simulink model "quadrotor_system_observer"  (R2022a)
settings: Solver=VariableStepAuto  StartTime=0.0  StopTime=70  RelTol=1e-3
values from neighbouring files (symbols this model uses):
  A1 = [-skew(Oc) ,eye(3),-skew(Vc),zeros(3),zeros(3,4) ... (first row only)    [controllerLinearizedSystemScript.m]
  B1 = [[0;0;0],zeros(3) ... (first row only)    [controllerLinearizedSystemScript.m]
  C1 = [eye(3), zeros(3), zeros(3), zeros(3), zeros(3,4) ... (first row only)    [controllerLinearizedSystemScript.m]
  K1 = lqr(A1,B1,Q1,R1,0)    [controllerLinearizedSystemScript.m]
undefined symbols (not defined in the file or in its folder): L
libraries: robotcorelib x1, uavutilslib x1
settings Model: PacingRate=4  Creator=Lenovo  LastModifiedBy=FLKU

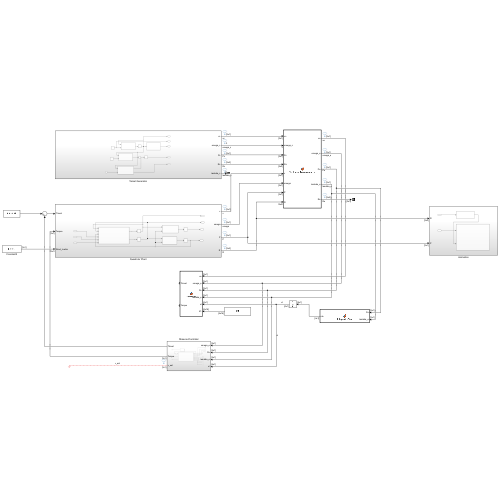
[thumbnail: Simulink's stored preview of the top-level diagram]
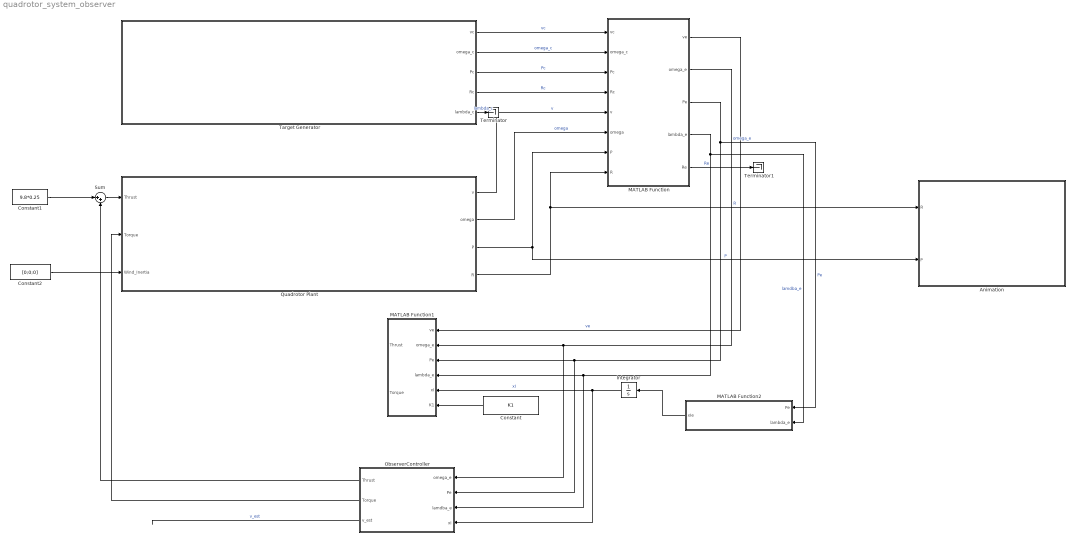
== system quadrotor_system_observer ==
  Animation : Subsystem
  Constant : Constant  Value=K1
  Constant1 : Constant  Value=9.8*0.25
  Constant2 : Constant  Value=[0;0;0]  VectorParams1D=off  SampleTime=-1
  Integrator : Integrator
  MATLAB Function : MATLAB Function  TreatAsAtomicUnit=on
  MATLAB Function1 : MATLAB Function  TreatAsAtomicUnit=on
  MATLAB Function2 : MATLAB Function  TreatAsAtomicUnit=on
  ObserverController : Subsystem
  Quadrotor Plant : Subsystem
  Sum : Sum  Inputs=|++
  Target Generator : Subsystem
  Terminator : Terminator
  Terminator1 : Terminator
  wires:
  Target Generator/1(vc) -> MATLAB Function/1(vc)  "vc"
  Target Generator/2(omega_c) -> MATLAB Function/2(omega_c)  "omega_c"
  Target Generator/3(Pc) -> MATLAB Function/3(Pc)  "Pc"
  Target Generator/4(Rc) -> MATLAB Function/4(Rc)  "Rc"
  Quadrotor Plant/4(R) -> MATLAB Function/8(R), Animation/1(R)  "R"
  Quadrotor Plant/3(P) -> Animation/2(P), MATLAB Function/7(P)  "P"
  Quadrotor Plant/2(omega) -> MATLAB Function/6(omega)  "omega"
  Quadrotor Plant/1(v) -> MATLAB Function/5(v)  "v"
  MATLAB Function/4(lambda_e) -> ObserverController/3(lamdba_e), MATLAB Function1/4(lambda_e), MATLAB Function2/2(lambda_e)  "lamdba_e"
  MATLAB Function/3(Pe) -> MATLAB Function1/3(Pe), ObserverController/2(Pe), MATLAB Function2/1(Pe)  "Pe"
  MATLAB Function/2(omega_e) -> MATLAB Function1/2(omega_e), ObserverController/1(omega_e)  "omega_e"
  MATLAB Function/1(ve) -> MATLAB Function1/1(ve)  "ve"
  Target Generator/5(lambda_c) -> Terminator/1  "lambda_c"
  Constant/1 -> MATLAB Function1/6(K1)
  Sum/1 -> Quadrotor Plant/1(Thrust)
  Constant1/1 -> Sum/1
  Constant2/1 -> Quadrotor Plant/3(Wind_Inertia)
  MATLAB Function2/1(xIe) -> Integrator/1
  Integrator/1 -> ObserverController/4(xI), MATLAB Function1/5(xI)  "xI"
  MATLAB Function/5(Re) -> Terminator1/1  "Re"
  ObserverController/3(v_est) -> ?  "v_est"
  ObserverController/1(Thrust) -> Sum/2
  ObserverController/2(Torque) -> Quadrotor Plant/2(Torque)

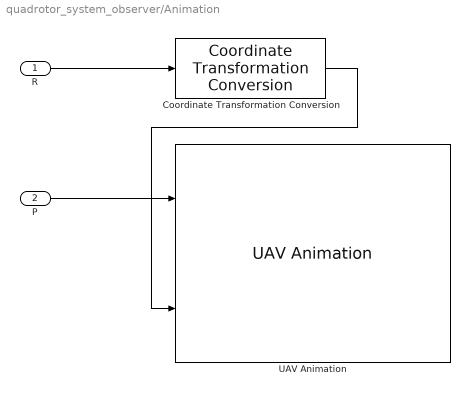
== system quadrotor_system_observer/Animation ==
  R : Inport
  P : Inport  Port=2
  Coordinate Transformation Conversion : robotcorelib/Coordinate Transformation Conversion  InputRepresentation=Rotation Matrix  InputEulerSequence=ZYX  ShowTrVecInputPort=on  OutputRepresentation=Quaternion  OutputEulerSequence=ZYX  ShowTrVecOutputPort=on  SimulateUsing=Interpreted execution
      settings: SourceProductBaseCode=RO,NV,RR,UV
  UAV Animation : uavutilslib/UAV Animation  UAVType=Multirotor  UAVSize=1  InertialZDirection=Down  SampleTime=-1
      settings: SourceProductBaseCode=UV
  wires:
  Coordinate Transformation Conversion/1 -> UAV Animation/2
  P/1 -> UAV Animation/1
  R/1 -> Coordinate Transformation Conversion/1

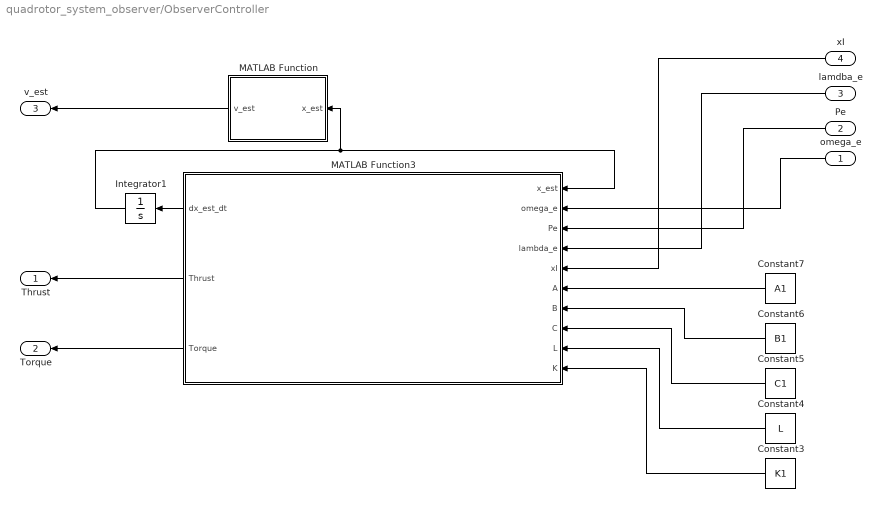
== system quadrotor_system_observer/ObserverController ==
  omega_e : Inport
  Pe : Inport  Port=2
  lamdba_e : Inport  Port=3
  xI : Inport  Port=4
  Constant3 : Constant  Value=K1
  Constant4 : Constant  Value=L
  Constant5 : Constant  Value=C1
  Constant6 : Constant  Value=B1
  Constant7 : Constant  Value=A1
  Integrator1 : Integrator  InitialCondition=zeros(16,1)
  MATLAB Function : MATLAB Function  TreatAsAtomicUnit=on
  MATLAB Function3 : MATLAB Function  TreatAsAtomicUnit=on
  Thrust : Outport
  Torque : Outport  Port=2
  v_est : Outport  Port=3
  wires:
  Constant7/1 -> MATLAB Function3/6(A)
  MATLAB Function3/3(Torque) -> Torque/1
  Constant4/1 -> MATLAB Function3/9(L)
  Integrator1/1 -> MATLAB Function/1(x_est), MATLAB Function3/1(x_est)
  Constant6/1 -> MATLAB Function3/7(B)
  Constant3/1 -> MATLAB Function3/10(K)
  MATLAB Function3/1(dx_est_dt) -> Integrator1/1
  Constant5/1 -> MATLAB Function3/8(C)
  MATLAB Function3/2(Thrust) -> Thrust/1
  xI/1 -> MATLAB Function3/5(xI)
  omega_e/1 -> MATLAB Function3/2(omega_e)
  Pe/1 -> MATLAB Function3/3(Pe)
  lamdba_e/1 -> MATLAB Function3/4(lambda_e)
  MATLAB Function/1(v_est) -> v_est/1

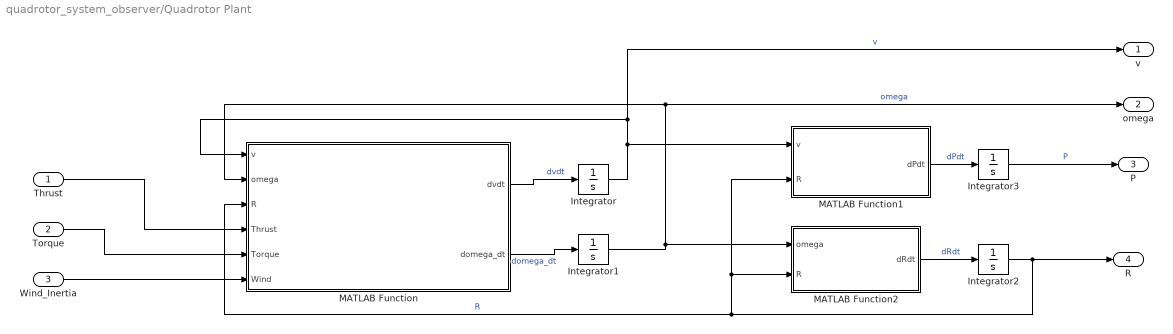
== system quadrotor_system_observer/Quadrotor Plant ==
  Thrust : Inport
  Torque : Inport  Port=2
  Wind_Inertia : Inport  Port=3
  Integrator : Integrator  InitialCondition=[0;0;0]
  Integrator1 : Integrator  InitialCondition=[0;0;0]
  Integrator2 : Integrator  InitialCondition=eye(3)
  Integrator3 : Integrator  InitialCondition=[0;0;0]
  MATLAB Function : MATLAB Function  TreatAsAtomicUnit=on
  MATLAB Function1 : MATLAB Function  TreatAsAtomicUnit=on
  MATLAB Function2 : MATLAB Function  TreatAsAtomicUnit=on
  v : Outport
  omega : Outport  Port=2
  P : Outport  Port=3
  R : Outport  Port=4
  wires:
  Integrator2/1 -> R/1, MATLAB Function/3(R), MATLAB Function2/2(R), MATLAB Function1/2(R)  "R"
  MATLAB Function/1(dvdt) -> Integrator/1  "dvdt"
  Integrator1/1 -> MATLAB Function2/1(omega), MATLAB Function/2(omega), omega/1  "omega"
  MATLAB Function/2(domega_dt) -> Integrator1/1  "domega_dt"
  Thrust/1 -> MATLAB Function/4(Thrust)
  MATLAB Function1/1(dPdt) -> Integrator3/1  "dPdt"
  Integrator3/1 -> P/1  "P"
  MATLAB Function2/1(dRdt) -> Integrator2/1  "dRdt"
  Integrator/1 -> v/1, MATLAB Function/1(v), MATLAB Function1/1(v)  "v"
  Torque/1 -> MATLAB Function/5(Torque)
  Wind_Inertia/1 -> MATLAB Function/6(Wind)

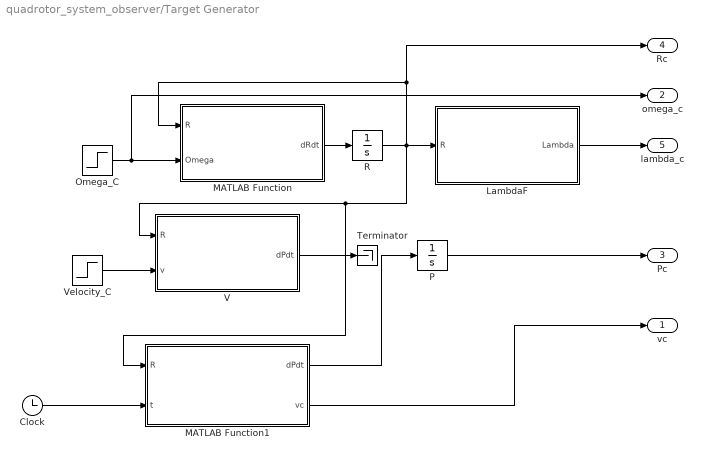
== system quadrotor_system_observer/Target Generator ==
  Clock : Clock
  LambdaF : MATLAB Function  TreatAsAtomicUnit=on
  MATLAB Function : MATLAB Function  TreatAsAtomicUnit=on
  MATLAB Function1 : MATLAB Function  TreatAsAtomicUnit=on
  Omega_C : Step  Time=0  Before=[0;0;0]  After=[0;0;0]  SampleTime=0
  P : Integrator  InitialCondition=[0;0;0]
  R : Integrator  InitialCondition=eye(3)
  Terminator : Terminator
  V : MATLAB Function  TreatAsAtomicUnit=on
  Velocity_C : Step  Time=0  Before=[0;0;0]  After=[2;0;0]  SampleTime=0
  vc : Outport
  omega_c : Outport  Port=2
  Pc : Outport  Port=3
  Rc : Outport  Port=4
  lambda_c : Outport  Port=5
  wires:
  LambdaF/1(Lambda) -> lambda_c/1
  P/1 -> Pc/1
  MATLAB Function/1(dRdt) -> R/1
  R/1 -> MATLAB Function/1(R), Rc/1, MATLAB Function1/1(R), V/1(R), LambdaF/1(R)
  Velocity_C/1 -> V/2(v)
  Omega_C/1 -> omega_c/1, MATLAB Function/2(Omega)
  Clock/1 -> MATLAB Function1/2(t)
  MATLAB Function1/1(dPdt) -> P/1
  MATLAB Function1/2(vc) -> vc/1
  V/1(dPdt) -> Terminator/1

== matlab function quadrotor_system_observer/MATLAB Function2 ==
  data: Pe input; xIe output; lambda_e input
function xIe = IntegrationVar(Pe,lambda_e)

xIe = [Pe;lambda_e(3)];

== matlab function quadrotor_system_observer/ObserverController/MATLAB Function3 ==
  data: x_est input; omega_e input; dx_est_dt output; Pe input; lambda_e input; xI input; A input; B input; C input; L input; K input; Thrust output; Torque output
function [dx_est_dt,Thrust,Torque]   = observer_controller(x_est,omega_e,Pe,lambda_e,xI,A,B,C,L,K)
%% controller
u = -K*x_est;
Thrust=u(1);
Torque=u(2:4);
%% observer
y=[Pe;lambda_e;omega_e;xI];
dx_est_dt = (A-L*C)*x_est+L*y+B*u;
end

== matlab function quadrotor_system_observer/Target Generator/MATLAB Function1 ==
  data: R input; t input; dPdt output; vc output
function [dPdt,vc] = GenRecTrajVc(R,t)
v = 0.5;
vc = [0;0;0];
if t>5
    vc = [v;0;0];
end
if t>15
    vc = [0;0;0];
end
if t>20
    vc = [0;v;0];
end
if t>30
    vc = [0;0;0];
end
if t>35
    vc = [-v;0;0];
end
if t>45
    vc = [0;0;0];
end
if t>50
    vc = [0;-v;0];
end
dPdt = R*vc;
end

== matlab function quadrotor_system_observer/ObserverController/MATLAB Function ==
  data: x_est input; v_est output
function v_est = chooseVEstima(x_est)

v_est = x_est(4:6);

== matlab function quadrotor_system_observer/Quadrotor Plant/MATLAB Function1 ==
  data: v input; dPdt output; R input
function dPdt = TranslationalKinematics(v,R)
dPdt = R*v;

== matlab function quadrotor_system_observer/Quadrotor Plant/MATLAB Function ==
  data: v input; omega input; R input; Thrust input; dvdt output; Torque input; domega_dt output; Wind input
function [dvdt, domega_dt] = Dynamics(v,omega,R,Thrust, Torque, Wind)
g = 9.807;
m = 0.24;
f_B = [0;0;-Thrust] + transpose(R) * [0;0;m*g] + transpose(R) * Wind;
I_B = diag([1e-4,1e-4,1e-3]);

dvdt = -skew(omega) * v + 1/m * f_B;
domega_dt = -(I_B^-1) * skew(omega) * I_B * omega + (I_B^-1) * Torque;
end

== matlab function quadrotor_system_observer/Quadrotor Plant/MATLAB Function2 ==
  data: omega input; dRdt output; R input
function dRdt = RotationalKinematics(omega,R)
dRdt = R*skew(omega);

== matlab function quadrotor_system_observer/Target Generator/V ==
  data: R input; dPdt output; v input
function dPdt = CompdPdt(R,v)
dPdt=R*v;
end

== matlab function quadrotor_system_observer/MATLAB Function ==
  data: vc input; ve output; omega_c input; Pc input; Rc input; v input; omega input; P input; R input; omega_e output; Pe output; lambda_e output; Re output
function [ve,omega_e,Pe, lambda_e, Re] = NonLinearTransformation(vc,omega_c,Pc,Rc, v,omega,P,R)
ve = v - vc;
omega_e = omega - omega_c;
% Pe = transpose(R) * (P-Pc);
Pe = P - Pc;
Re = R * Rc';
lambda_e = arg1(Re);

== matlab function quadrotor_system_observer/MATLAB Function1 ==
  data: ve input; Thrust output; omega_e input; Pe input; lambda_e input; xI input; Torque output; K1 input
function [Thrust, Torque] = Controller(ve,omega_e, Pe, lambda_e, xI, K1)
x = [Pe; ve; lambda_e;omega_e;xI];
u = -K1*x;

Thrust = u(1);
Torque = u(2:4);

== matlab function quadrotor_system_observer/Target Generator/LambdaF ==
  data: R input; Lambda output
function Lambda = R_to_Lambda(R)

Lambda = arg(R);

end

== matlab function quadrotor_system_observer/Target Generator/MATLAB Function ==
  data: R input; dRdt output; Omega input
function dRdt = CompdRdt(R,Omega)
dRdt=R*skew(Omega);
end
